simulink model "ME416_Autonomy_Model_Rollback2"  (R2025b)
settings: Solver=FixedStepAuto  StartTime=0.0  StopTime=240  RelTol=1e-3  EnableMultiTasking=on
PreLoadFcn:
  | driveparam
values from neighbouring files (symbols this model uses):
  alpha_w = 0.7    [driveparam.m]
  beta = Ts / (Ts + tau)    (= 0.166666666667)    [driveparam.m]
  enable_cmd = 1    [driveparam.m]
  estop_cmd = 0    [driveparam.m]
  K_lqr_w = dlqr(Ad_w, Bd_w, Qw, Rw)    [driveparam.m]
  L = 0.15    [driveparam.m]
  N = 4400    [driveparam.m]
  Nbar_lqr_w = (1 - Ad_w)/Bd_w + K_lqr_w    [driveparam.m]
  r = 0.03    [driveparam.m]
  Ts = 0.01    [driveparam.m]
  v_ref_cmd = 0    [driveparam.m]
  w_ref_cmd = 0.1    [driveparam.m]
undefined symbols (not defined in the file or in its folder): DiscIntNeverNeededParam, dspblkCoreblockFVToolHelper, gcbh
libraries: raspberrypiBasiclib x22, simulink x21, raspberrypiCommlib x19, slpidlib x2
(part 2 of 3)

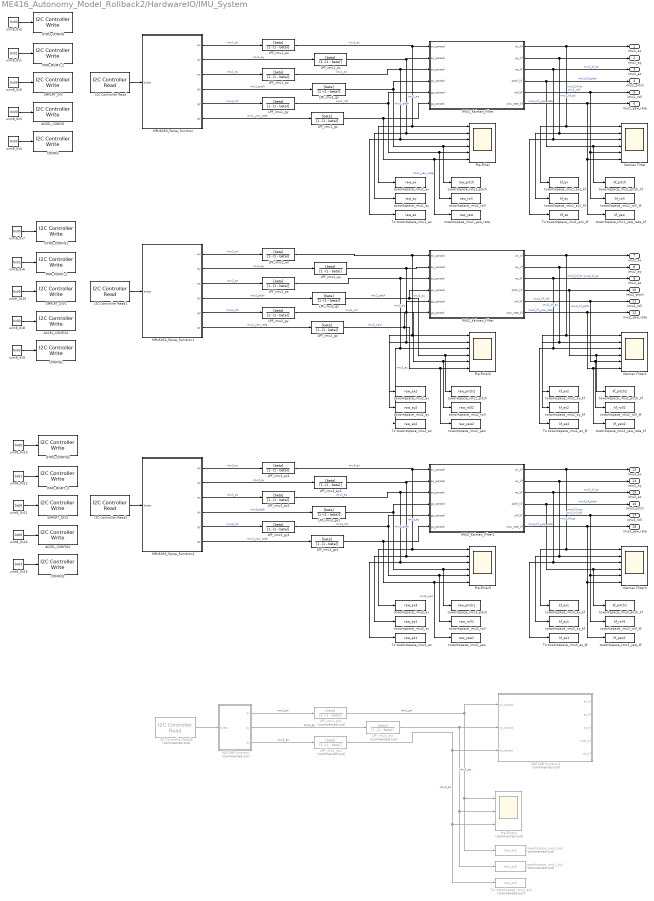
== system ME416_Autonomy_Model_Rollback2/HardwareIO/IMU_System ==
  ACCEL_CONFIG : raspberrypiCommlib/I2C Controller Write  BoardProperty=Pi 4 Model B  I2CModule=1  Mode=Master  SlaveAddress=0x68  SlaveByteOrder=BigEndian  Direction=Transmitter  RegisterAddressMode=on  RegisterAddress=0x1C  SlaveDataType=uint8  DataLength=1  NoAck=off  RepeatedStart=off  OutputStatus=off
  ACCEL_CONFIG1 : raspberrypiCommlib/I2C Controller Write  BoardProperty=Pi 4 Model B  I2CModule=0  Mode=Master  SlaveAddress=0x68  SlaveByteOrder=BigEndian  Direction=Transmitter  RegisterAddressMode=on  RegisterAddress=0x1C  SlaveDataType=uint8  DataLength=1  NoAck=off  RepeatedStart=off  OutputStatus=off
  ACCEL_CONFIG2 : raspberrypiCommlib/I2C Controller Write  BoardProperty=Pi 4 Model B  I2CModule=0  Mode=Master  SlaveAddress=0x69  SlaveByteOrder=BigEndian  Direction=Transmitter  RegisterAddressMode=on  RegisterAddress=0x1C  SlaveDataType=uint8  DataLength=1  NoAck=off  RepeatedStart=off  OutputStatus=off
  CONFIG : raspberrypiCommlib/I2C Controller Write  BoardProperty=Pi 4 Model B  I2CModule=1  Mode=Master  SlaveAddress=0x68  SlaveByteOrder=BigEndian  Direction=Transmitter  RegisterAddressMode=on  RegisterAddress=0x1A  SlaveDataType=uint8  DataLength=1  NoAck=off  RepeatedStart=off  OutputStatus=off
  CONFIG1 : raspberrypiCommlib/I2C Controller Write  BoardProperty=Pi 4 Model B  I2CModule=0  Mode=Master  SlaveAddress=0x68  SlaveByteOrder=BigEndian  Direction=Transmitter  RegisterAddressMode=on  RegisterAddress=0x1A  SlaveDataType=uint8  DataLength=1  NoAck=off  RepeatedStart=off  OutputStatus=off
  CONFIG2 : raspberrypiCommlib/I2C Controller Write  BoardProperty=Pi 4 Model B  I2CModule=0  Mode=Master  SlaveAddress=0x69  SlaveByteOrder=BigEndian  Direction=Transmitter  RegisterAddressMode=on  RegisterAddress=0x1A  SlaveDataType=uint8  DataLength=1  NoAck=off  RepeatedStart=off  OutputStatus=off
  GYRO_CONFIG : raspberrypiCommlib/I2C Controller Write  BoardProperty=Pi 4 Model B  I2CModule=1  Mode=Master  SlaveAddress=0x68  SlaveByteOrder=BigEndian  Direction=Transmitter  RegisterAddressMode=on  RegisterAddress=0x1B  SlaveDataType=uint8  DataLength=1  NoAck=off  RepeatedStart=off  OutputStatus=off
  GYRO_CONFIG1 : raspberrypiCommlib/I2C Controller Write  BoardProperty=Pi 4 Model B  I2CModule=0  Mode=Master  SlaveAddress=0x68  SlaveByteOrder=BigEndian  Direction=Transmitter  RegisterAddressMode=on  RegisterAddress=0x1B  SlaveDataType=uint8  DataLength=1  NoAck=off  RepeatedStart=off  OutputStatus=off
  GYRO_CONFIG2 : raspberrypiCommlib/I2C Controller Write  BoardProperty=Pi 4 Model B  I2CModule=0  Mode=Master  SlaveAddress=0x69  SlaveByteOrder=BigEndian  Direction=Transmitter  RegisterAddressMode=on  RegisterAddress=0x1B  SlaveDataType=uint8  DataLength=1  NoAck=off  RepeatedStart=off  OutputStatus=off
  I2C Controller Read : raspberrypiCommlib/I2C Controller Read  BoardProperty=Pi 4 Model B  I2CModule=1  Mode=Master  SlaveAddress=0x68  SlaveByteOrder=BigEndian  Direction=Receiver  RegisterAddressMode=on  RegisterAddress=0x3B  SlaveDataType=uint8  DataLength=14  NoAck=off  RepeatedStart=off  OutputStatus=off  SampleTime=0.01
  I2C Controller Read1 : raspberrypiCommlib/I2C Controller Read  BoardProperty=Pi 4 Model B  I2CModule=0  Mode=Master  SlaveAddress=0x68  SlaveByteOrder=BigEndian  Direction=Receiver  RegisterAddressMode=on  RegisterAddress=0x3B  SlaveDataType=uint8  DataLength=14  NoAck=off  RepeatedStart=off  OutputStatus=off  SampleTime=0.01
  I2C Controller Read2 : raspberrypiCommlib/I2C Controller Read  BoardProperty=Pi 4 Model B  I2CModule=0  Mode=Master  SlaveAddress=0x69  SlaveByteOrder=BigEndian  Direction=Receiver  RegisterAddressMode=on  RegisterAddress=0x3B  SlaveDataType=uint8  DataLength=14  NoAck=off  RepeatedStart=off  OutputStatus=off  SampleTime=0.01
  I2C Controller Read3 : raspberrypiCommlib/I2C Controller Read  Commented=on  BoardProperty=Pi 4 Model B  I2CModule=1  Mode=Master  SlaveAddress=0x1C  SlaveByteOrder=BigEndian  Direction=Receiver  RegisterAddressMode=on  RegisterAddress=0x01  SlaveDataType=uint8  DataLength=6  NoAck=off  RepeatedStart=off  OutputStatus=off  SampleTime=0.01
  IMU1_Kalman_Filter : MATLAB Function  TreatAsAtomicUnit=on
  IMU2_Kalman_Filter : MATLAB Function  TreatAsAtomicUnit=on
  IMU2_Kalman_Filter1 : MATLAB Function  TreatAsAtomicUnit=on
  Kalman Filter : Scope  NumInputPorts=6
      settings: ActiveDisplayYMinimum=-0.15082916961218429  ActiveDisplayYMaximum=0.016758796623576027
  Kalman Filter2 : Scope  NumInputPorts=6
      settings: ActiveDisplayYMinimum=-0.15082916961218429  ActiveDisplayYMaximum=0.016758796623576027  DataLoggingVariableName=ScopeData6
  Kalman Filter3 : Scope  NumInputPorts=6
      settings: ActiveDisplayYMinimum=-0.15082916961218429  ActiveDisplayYMaximum=0.016758796623576027  DataLoggingVariableName=ScopeData11
  LPF_imu1_ax : DiscreteTransferFcn  LoadFcn=dspblkCoreblockFVToolHelper(gcbh,'load');  Numerator=[beta]  Denominator=[1 -(1 - beta)]  SampleTime=Ts
      settings: CopyFcn=dspblkCoreblockFVToolHelper(gcbh,'copy');  DeleteFcn=dspblkCoreblockFVToolHelper(gcbh,'close');  ModelCloseFcn=dspblkCoreblockFVToolHelper(gcbh,'close');  PreSaveFcn=dspblkCoreblockFVToolHelper(gcbh,'presave');  PostSaveFcn=dspblkCoreblockFVToolHelper(gcbh,'postsave');  CloseFcn=dspblkCoreblockFVToolHelper(gcbh,'close');
  LPF_imu1_ax1 : DiscreteTransferFcn  Commented=on  LoadFcn=dspblkCoreblockFVToolHelper(gcbh,'load');  Numerator=[beta]  Denominator=[1 -(1 - beta)]  SampleTime=Ts
      settings: CopyFcn=dspblkCoreblockFVToolHelper(gcbh,'copy');  DeleteFcn=dspblkCoreblockFVToolHelper(gcbh,'close');  ModelCloseFcn=dspblkCoreblockFVToolHelper(gcbh,'close');  PreSaveFcn=dspblkCoreblockFVToolHelper(gcbh,'presave');  PostSaveFcn=dspblkCoreblockFVToolHelper(gcbh,'postsave');  CloseFcn=dspblkCoreblockFVToolHelper(gcbh,'close');
  LPF_imu1_ay : DiscreteTransferFcn  LoadFcn=dspblkCoreblockFVToolHelper(gcbh,'load');  Numerator=[beta]  Denominator=[1 -(1 - beta)]  SampleTime=Ts
      settings: CopyFcn=dspblkCoreblockFVToolHelper(gcbh,'copy');  DeleteFcn=dspblkCoreblockFVToolHelper(gcbh,'close');  ModelCloseFcn=dspblkCoreblockFVToolHelper(gcbh,'close');  PreSaveFcn=dspblkCoreblockFVToolHelper(gcbh,'presave');  PostSaveFcn=dspblkCoreblockFVToolHelper(gcbh,'postsave');  CloseFcn=dspblkCoreblockFVToolHelper(gcbh,'close');
  LPF_imu1_ay1 : DiscreteTransferFcn  Commented=on  LoadFcn=dspblkCoreblockFVToolHelper(gcbh,'load');  Numerator=[beta]  Denominator=[1 -(1 - beta)]  SampleTime=Ts
      settings: CopyFcn=dspblkCoreblockFVToolHelper(gcbh,'copy');  DeleteFcn=dspblkCoreblockFVToolHelper(gcbh,'close');  ModelCloseFcn=dspblkCoreblockFVToolHelper(gcbh,'close');  PreSaveFcn=dspblkCoreblockFVToolHelper(gcbh,'presave');  PostSaveFcn=dspblkCoreblockFVToolHelper(gcbh,'postsave');  CloseFcn=dspblkCoreblockFVToolHelper(gcbh,'close');
  LPF_imu1_az : DiscreteTransferFcn  LoadFcn=dspblkCoreblockFVToolHelper(gcbh,'load');  Numerator=[beta]  Denominator=[1 -(1 - beta)]  SampleTime=Ts
      settings: CopyFcn=dspblkCoreblockFVToolHelper(gcbh,'copy');  DeleteFcn=dspblkCoreblockFVToolHelper(gcbh,'close');  ModelCloseFcn=dspblkCoreblockFVToolHelper(gcbh,'close');  PreSaveFcn=dspblkCoreblockFVToolHelper(gcbh,'presave');  PostSaveFcn=dspblkCoreblockFVToolHelper(gcbh,'postsave');  CloseFcn=dspblkCoreblockFVToolHelper(gcbh,'close');
  LPF_imu1_az1 : DiscreteTransferFcn  Commented=on  LoadFcn=dspblkCoreblockFVToolHelper(gcbh,'load');  Numerator=[beta]  Denominator=[1 -(1 - beta)]  SampleTime=Ts
      settings: CopyFcn=dspblkCoreblockFVToolHelper(gcbh,'copy');  DeleteFcn=dspblkCoreblockFVToolHelper(gcbh,'close');  ModelCloseFcn=dspblkCoreblockFVToolHelper(gcbh,'close');  PreSaveFcn=dspblkCoreblockFVToolHelper(gcbh,'presave');  PostSaveFcn=dspblkCoreblockFVToolHelper(gcbh,'postsave');  CloseFcn=dspblkCoreblockFVToolHelper(gcbh,'close');
  LPF_imu1_gx : DiscreteTransferFcn  LoadFcn=dspblkCoreblockFVToolHelper(gcbh,'load');  Numerator=[beta]  Denominator=[1 -(1 - beta)]  SampleTime=Ts
      settings: CopyFcn=dspblkCoreblockFVToolHelper(gcbh,'copy');  DeleteFcn=dspblkCoreblockFVToolHelper(gcbh,'close');  ModelCloseFcn=dspblkCoreblockFVToolHelper(gcbh,'close');  PreSaveFcn=dspblkCoreblockFVToolHelper(gcbh,'presave');  PostSaveFcn=dspblkCoreblockFVToolHelper(gcbh,'postsave');  CloseFcn=dspblkCoreblockFVToolHelper(gcbh,'close');
  LPF_imu1_gy : DiscreteTransferFcn  LoadFcn=dspblkCoreblockFVToolHelper(gcbh,'load');  Numerator=[beta]  Denominator=[1 -(1 - beta)]  SampleTime=Ts
      settings: CopyFcn=dspblkCoreblockFVToolHelper(gcbh,'copy');  DeleteFcn=dspblkCoreblockFVToolHelper(gcbh,'close');  ModelCloseFcn=dspblkCoreblockFVToolHelper(gcbh,'close');  PreSaveFcn=dspblkCoreblockFVToolHelper(gcbh,'presave');  PostSaveFcn=dspblkCoreblockFVToolHelper(gcbh,'postsave');  CloseFcn=dspblkCoreblockFVToolHelper(gcbh,'close');
  LPF_imu1_gz : DiscreteTransferFcn  LoadFcn=dspblkCoreblockFVToolHelper(gcbh,'load');  Numerator=[beta]  Denominator=[1 -(1 - beta)]  SampleTime=Ts
      settings: CopyFcn=dspblkCoreblockFVToolHelper(gcbh,'copy');  DeleteFcn=dspblkCoreblockFVToolHelper(gcbh,'close');  ModelCloseFcn=dspblkCoreblockFVToolHelper(gcbh,'close');  PreSaveFcn=dspblkCoreblockFVToolHelper(gcbh,'presave');  PostSaveFcn=dspblkCoreblockFVToolHelper(gcbh,'postsave');  CloseFcn=dspblkCoreblockFVToolHelper(gcbh,'close');
  LPF_imu2_ax : DiscreteTransferFcn  LoadFcn=dspblkCoreblockFVToolHelper(gcbh,'load');  Numerator=[beta]  Denominator=[1 -(1 - beta)]  SampleTime=Ts
      settings: CopyFcn=dspblkCoreblockFVToolHelper(gcbh,'copy');  DeleteFcn=dspblkCoreblockFVToolHelper(gcbh,'close');  ModelCloseFcn=dspblkCoreblockFVToolHelper(gcbh,'close');  PreSaveFcn=dspblkCoreblockFVToolHelper(gcbh,'presave');  PostSaveFcn=dspblkCoreblockFVToolHelper(gcbh,'postsave');  CloseFcn=dspblkCoreblockFVToolHelper(gcbh,'close');
  LPF_imu2_ay : DiscreteTransferFcn  LoadFcn=dspblkCoreblockFVToolHelper(gcbh,'load');  Numerator=[beta]  Denominator=[1 -(1 - beta)]  SampleTime=Ts
      settings: CopyFcn=dspblkCoreblockFVToolHelper(gcbh,'copy');  DeleteFcn=dspblkCoreblockFVToolHelper(gcbh,'close');  ModelCloseFcn=dspblkCoreblockFVToolHelper(gcbh,'close');  PreSaveFcn=dspblkCoreblockFVToolHelper(gcbh,'presave');  PostSaveFcn=dspblkCoreblockFVToolHelper(gcbh,'postsave');  CloseFcn=dspblkCoreblockFVToolHelper(gcbh,'close');
  LPF_imu2_az : DiscreteTransferFcn  LoadFcn=dspblkCoreblockFVToolHelper(gcbh,'load');  Numerator=[beta]  Denominator=[1 -(1 - beta)]  SampleTime=Ts
      settings: CopyFcn=dspblkCoreblockFVToolHelper(gcbh,'copy');  DeleteFcn=dspblkCoreblockFVToolHelper(gcbh,'close');  ModelCloseFcn=dspblkCoreblockFVToolHelper(gcbh,'close');  PreSaveFcn=dspblkCoreblockFVToolHelper(gcbh,'presave');  PostSaveFcn=dspblkCoreblockFVToolHelper(gcbh,'postsave');  CloseFcn=dspblkCoreblockFVToolHelper(gcbh,'close');
  LPF_imu2_gx : DiscreteTransferFcn  LoadFcn=dspblkCoreblockFVToolHelper(gcbh,'load');  Numerator=[beta]  Denominator=[1 -(1 - beta)]  SampleTime=Ts
      settings: CopyFcn=dspblkCoreblockFVToolHelper(gcbh,'copy');  DeleteFcn=dspblkCoreblockFVToolHelper(gcbh,'close');  ModelCloseFcn=dspblkCoreblockFVToolHelper(gcbh,'close');  PreSaveFcn=dspblkCoreblockFVToolHelper(gcbh,'presave');  PostSaveFcn=dspblkCoreblockFVToolHelper(gcbh,'postsave');  CloseFcn=dspblkCoreblockFVToolHelper(gcbh,'close');
  LPF_imu2_gy : DiscreteTransferFcn  LoadFcn=dspblkCoreblockFVToolHelper(gcbh,'load');  Numerator=[beta]  Denominator=[1 -(1 - beta)]  SampleTime=Ts
      settings: CopyFcn=dspblkCoreblockFVToolHelper(gcbh,'copy');  DeleteFcn=dspblkCoreblockFVToolHelper(gcbh,'close');  ModelCloseFcn=dspblkCoreblockFVToolHelper(gcbh,'close');  PreSaveFcn=dspblkCoreblockFVToolHelper(gcbh,'presave');  PostSaveFcn=dspblkCoreblockFVToolHelper(gcbh,'postsave');  CloseFcn=dspblkCoreblockFVToolHelper(gcbh,'close');
  LPF_imu2_gz : DiscreteTransferFcn  LoadFcn=dspblkCoreblockFVToolHelper(gcbh,'load');  Numerator=[beta]  Denominator=[1 -(1 - beta)]  SampleTime=Ts
      settings: CopyFcn=dspblkCoreblockFVToolHelper(gcbh,'copy');  DeleteFcn=dspblkCoreblockFVToolHelper(gcbh,'close');  ModelCloseFcn=dspblkCoreblockFVToolHelper(gcbh,'close');  PreSaveFcn=dspblkCoreblockFVToolHelper(gcbh,'presave');  PostSaveFcn=dspblkCoreblockFVToolHelper(gcbh,'postsave');  CloseFcn=dspblkCoreblockFVToolHelper(gcbh,'close');
  LPF_imu3_ax1 : DiscreteTransferFcn  LoadFcn=dspblkCoreblockFVToolHelper(gcbh,'load');  Numerator=[beta]  Denominator=[1 -(1 - beta)]  SampleTime=Ts
      settings: CopyFcn=dspblkCoreblockFVToolHelper(gcbh,'copy');  DeleteFcn=dspblkCoreblockFVToolHelper(gcbh,'close');  ModelCloseFcn=dspblkCoreblockFVToolHelper(gcbh,'close');  PreSaveFcn=dspblkCoreblockFVToolHelper(gcbh,'presave');  PostSaveFcn=dspblkCoreblockFVToolHelper(gcbh,'postsave');  CloseFcn=dspblkCoreblockFVToolHelper(gcbh,'close');
  LPF_imu3_ay1 : DiscreteTransferFcn  LoadFcn=dspblkCoreblockFVToolHelper(gcbh,'load');  Numerator=[beta]  Denominator=[1 -(1 - beta)]  SampleTime=Ts
      settings: CopyFcn=dspblkCoreblockFVToolHelper(gcbh,'copy');  DeleteFcn=dspblkCoreblockFVToolHelper(gcbh,'close');  ModelCloseFcn=dspblkCoreblockFVToolHelper(gcbh,'close');  PreSaveFcn=dspblkCoreblockFVToolHelper(gcbh,'presave');  PostSaveFcn=dspblkCoreblockFVToolHelper(gcbh,'postsave');  CloseFcn=dspblkCoreblockFVToolHelper(gcbh,'close');
  LPF_imu3_az1 : DiscreteTransferFcn  LoadFcn=dspblkCoreblockFVToolHelper(gcbh,'load');  Numerator=[beta]  Denominator=[1 -(1 - beta)]  SampleTime=Ts
      settings: CopyFcn=dspblkCoreblockFVToolHelper(gcbh,'copy');  DeleteFcn=dspblkCoreblockFVToolHelper(gcbh,'close');  ModelCloseFcn=dspblkCoreblockFVToolHelper(gcbh,'close');  PreSaveFcn=dspblkCoreblockFVToolHelper(gcbh,'presave');  PostSaveFcn=dspblkCoreblockFVToolHelper(gcbh,'postsave');  CloseFcn=dspblkCoreblockFVToolHelper(gcbh,'close');
  LPF_imu3_gx1 : DiscreteTransferFcn  LoadFcn=dspblkCoreblockFVToolHelper(gcbh,'load');  Numerator=[beta]  Denominator=[1 -(1 - beta)]  SampleTime=Ts
      settings: CopyFcn=dspblkCoreblockFVToolHelper(gcbh,'copy');  DeleteFcn=dspblkCoreblockFVToolHelper(gcbh,'close');  ModelCloseFcn=dspblkCoreblockFVToolHelper(gcbh,'close');  PreSaveFcn=dspblkCoreblockFVToolHelper(gcbh,'presave');  PostSaveFcn=dspblkCoreblockFVToolHelper(gcbh,'postsave');  CloseFcn=dspblkCoreblockFVToolHelper(gcbh,'close');
  LPF_imu3_gy1 : DiscreteTransferFcn  LoadFcn=dspblkCoreblockFVToolHelper(gcbh,'load');  Numerator=[beta]  Denominator=[1 -(1 - beta)]  SampleTime=Ts
      settings: CopyFcn=dspblkCoreblockFVToolHelper(gcbh,'copy');  DeleteFcn=dspblkCoreblockFVToolHelper(gcbh,'close');  ModelCloseFcn=dspblkCoreblockFVToolHelper(gcbh,'close');  PreSaveFcn=dspblkCoreblockFVToolHelper(gcbh,'presave');  PostSaveFcn=dspblkCoreblockFVToolHelper(gcbh,'postsave');  CloseFcn=dspblkCoreblockFVToolHelper(gcbh,'close');
  LPF_imu3_gz1 : DiscreteTransferFcn  LoadFcn=dspblkCoreblockFVToolHelper(gcbh,'load');  Numerator=[beta]  Denominator=[1 -(1 - beta)]  SampleTime=Ts
      settings: CopyFcn=dspblkCoreblockFVToolHelper(gcbh,'copy');  DeleteFcn=dspblkCoreblockFVToolHelper(gcbh,'close');  ModelCloseFcn=dspblkCoreblockFVToolHelper(gcbh,'close');  PreSaveFcn=dspblkCoreblockFVToolHelper(gcbh,'presave');  PostSaveFcn=dspblkCoreblockFVToolHelper(gcbh,'postsave');  CloseFcn=dspblkCoreblockFVToolHelper(gcbh,'close');
  MATLAB Function : MATLAB Function  Commented=on  TreatAsAtomicUnit=on
  MATLAB Function1 : MATLAB Function  Commented=on  TreatAsAtomicUnit=on
  MPU6050_Parse_Function : MATLAB Function  TreatAsAtomicUnit=on
  MPU6050_Parse_Function1 : MATLAB Function  TreatAsAtomicUnit=on
  MPU6050_Parse_Function2 : MATLAB Function  TreatAsAtomicUnit=on
  PWR_MGMT_1 : raspberrypiCommlib/I2C Controller Write  BoardProperty=Pi 4 Model B  I2CModule=1  Mode=Master  SlaveAddress=0x68  SlaveByteOrder=BigEndian  Direction=Transmitter  RegisterAddressMode=on  RegisterAddress=0x6B  SlaveDataType=uint8  DataLength=1  NoAck=off  RepeatedStart=off  OutputStatus=off
  PWR_MGMT_2 : raspberrypiCommlib/I2C Controller Write  BoardProperty=Pi 4 Model B  I2CModule=0  Mode=Master  SlaveAddress=0x68  SlaveByteOrder=BigEndian  Direction=Transmitter  RegisterAddressMode=on  RegisterAddress=0x6B  SlaveDataType=uint8  DataLength=1  NoAck=off  RepeatedStart=off  OutputStatus=off
  PWR_MGMT_3 : raspberrypiCommlib/I2C Controller Write  BoardProperty=Pi 4 Model B  I2CModule=0  Mode=Master  SlaveAddress=0x69  SlaveByteOrder=BigEndian  Direction=Transmitter  RegisterAddressMode=on  RegisterAddress=0x6B  SlaveDataType=uint8  DataLength=1  NoAck=off  RepeatedStart=off  OutputStatus=off
  Pre-Filter : Scope  NumInputPorts=6
      settings: ActiveDisplayYMinimum=-0.68608023128352935  ActiveDisplayYMaximum=0.076231136809281022  DataLoggingVariableName=ScopeData5
  Pre-Filter1 : Scope  Commented=on  NumInputPorts=3
      settings: ActiveDisplayYMinimum=-0.68608023128352935  ActiveDisplayYMaximum=0.076231136809281022  DataLoggingVariableName=ScopeData13
  Pre-Filter2 : Scope  NumInputPorts=6
      settings: ActiveDisplayYMinimum=-0.68608023128352935  ActiveDisplayYMaximum=0.076231136809281022  DataLoggingVariableName=ScopeData10
  Pre-Filter3 : Scope  NumInputPorts=6
      settings: ActiveDisplayYMinimum=-0.68608023128352935  ActiveDisplayYMaximum=0.076231136809281022  DataLoggingVariableName=ScopeData12
  SMPLRT_DIV : raspberrypiCommlib/I2C Controller Write  BoardProperty=Pi 4 Model B  I2CModule=1  Mode=Master  SlaveAddress=0x68  SlaveByteOrder=BigEndian  Direction=Transmitter  RegisterAddressMode=on  RegisterAddress=0x19  SlaveDataType=uint8  DataLength=1  NoAck=off  RepeatedStart=off  OutputStatus=off
  SMPLRT_DIV1 : raspberrypiCommlib/I2C Controller Write  BoardProperty=Pi 4 Model B  I2CModule=0  Mode=Master  SlaveAddress=0x68  SlaveByteOrder=BigEndian  Direction=Transmitter  RegisterAddressMode=on  RegisterAddress=0x19  SlaveDataType=uint8  DataLength=1  NoAck=off  RepeatedStart=off  OutputStatus=off
  SMPLRT_DIV2 : raspberrypiCommlib/I2C Controller Write  BoardProperty=Pi 4 Model B  I2CModule=0  Mode=Master  SlaveAddress=0x69  SlaveByteOrder=BigEndian  Direction=Transmitter  RegisterAddressMode=on  RegisterAddress=0x19  SlaveDataType=uint8  DataLength=1  NoAck=off  RepeatedStart=off  OutputStatus=off
  To toworkspace_imu1_az : ToWorkspace  VariableName=raw_az  SampleTime=-1
  To toworkspace_imu1_az1 : ToWorkspace  Commented=on  VariableName=raw_az3  SampleTime=-1
  To toworkspace_imu1_az1_kf : ToWorkspace  VariableName=kf_az  SampleTime=-1
  To toworkspace_imu2_az : ToWorkspace  VariableName=raw_az2  SampleTime=-1
  To toworkspace_imu2_az_kf : ToWorkspace  VariableName=kf_az2  SampleTime=-1
  To toworkspace_imu3_az : ToWorkspace  VariableName=raw_az1  SampleTime=-1
  To toworkspace_imu3_az_kf : ToWorkspace  VariableName=kf_az1  SampleTime=-1
  toworkspace_imu1_ax : ToWorkspace  VariableName=raw_ax  SampleTime=-1
  toworkspace_imu1_ax1 : ToWorkspace  Commented=on  VariableName=raw_ax1  SampleTime=-1
  toworkspace_imu1_ax1_kf : ToWorkspace  VariableName=kf_ax  SampleTime=-1
  toworkspace_imu1_ay : ToWorkspace  VariableName=raw_ay  SampleTime=-1
  toworkspace_imu1_ay1 : ToWorkspace  Commented=on  VariableName=raw_ay3  SampleTime=-1
  toworkspace_imu1_ay1_kf : ToWorkspace  VariableName=kf_ay  SampleTime=-1
  toworkspace_imu1_pitch : ToWorkspace  VariableName=raw_pitch  SampleTime=-1
  toworkspace_imu1_pitch_kf : ToWorkspace  VariableName=kf_pitch  SampleTime=-1
  toworkspace_imu1_roll : ToWorkspace  VariableName=raw_roll  SampleTime=-1
  toworkspace_imu1_roll_kf : ToWorkspace  VariableName=kf_roll  SampleTime=-1
  toworkspace_imu1_yaw_rate : ToWorkspace  VariableName=raw_yaw  SampleTime=-1
  toworkspace_imu1_yaw_rate_kf : ToWorkspace  VariableName=kf_yaw  SampleTime=-1
  toworkspace_imu2_ax : ToWorkspace  VariableName=raw_ax2  SampleTime=-1
  toworkspace_imu2_ax_kf : ToWorkspace  VariableName=kf_ax2  SampleTime=-1
  toworkspace_imu2_ay : ToWorkspace  VariableName=raw_ay2  SampleTime=-1
  toworkspace_imu2_ay_kf : ToWorkspace  VariableName=kf_ay2  SampleTime=-1
  toworkspace_imu2_pitch : ToWorkspace  VariableName=raw_pitch2  SampleTime=-1
  toworkspace_imu2_pitch_kf : ToWorkspace  VariableName=kf_pitch2  SampleTime=-1
  toworkspace_imu2_roll : ToWorkspace  VariableName=raw_roll2  SampleTime=-1
  toworkspace_imu2_roll_kf : ToWorkspace  VariableName=kf_roll2  SampleTime=-1
  toworkspace_imu2_yaw : ToWorkspace  VariableName=raw_yaw2  SampleTime=-1
  toworkspace_imu2_yaw_rate_kf : ToWorkspace  VariableName=kf_yaw2  SampleTime=-1
  toworkspace_imu3_ax : ToWorkspace  VariableName=raw_ax3  SampleTime=-1
  toworkspace_imu3_ax_kf : ToWorkspace  VariableName=kf_ax1  SampleTime=-1
  toworkspace_imu3_ay : ToWorkspace  VariableName=raw_ay1  SampleTime=-1
  toworkspace_imu3_ay_kf : ToWorkspace  VariableName=kf_ay1  SampleTime=-1
  toworkspace_imu3_pitch : ToWorkspace  VariableName=raw_pitch1  SampleTime=-1
  toworkspace_imu3_pitch_kf : ToWorkspace  VariableName=kf_pitch1  SampleTime=-1
  toworkspace_imu3_roll : ToWorkspace  VariableName=raw_roll1  SampleTime=-1
  toworkspace_imu3_roll_kf : ToWorkspace  VariableName=kf_roll1  SampleTime=-1
  toworkspace_imu3_yaw : ToWorkspace  VariableName=raw_yaw1  SampleTime=-1
  toworkspace_imu3_yaw_kf : ToWorkspace  VariableName=kf_yaw1  SampleTime=-1
  uint8_0x1 : Constant  Value=0x01  OutDataTypeStr=uint8
  uint8_0x10 : Constant  Value=0x09  OutDataTypeStr=uint8
  uint8_0x11 : Constant  Value=0x09  OutDataTypeStr=uint8
  uint8_0x12 : Constant  Value=0x01  OutDataTypeStr=uint8
  uint8_0x{2..3,7..8,13..14} (6 alike) : Constant  Value=0x00  OutDataTypeStr=uint8
  uint8_0x15 : Constant  Value=0x03  OutDataTypeStr=uint8
  uint8_0x4 : Constant  Value=0x03  OutDataTypeStr=uint8
  uint8_0x5 : Constant  Value=0x09  OutDataTypeStr=uint8
  uint8_0x6 : Constant  Value=0x01  OutDataTypeStr=uint8
  uint8_0x9 : Constant  Value=0x03  OutDataTypeStr=uint8
  imu1_ax : Outport
  imu1_ay : Outport  Port=2
  imu1_az : Outport  Port=3
  imu1_pitch : Outport  Port=4
  imu1_roll : Outport  Port=5
  imu1_yaw_rate : Outport  Port=6
  imu2_ax : Outport  Port=7
  imu2_ay : Outport  Port=8
  imu2_az : Outport  Port=9
  imu2_pitch : Outport  Port=10
  imu2_roll : Outport  Port=11
  imu2_yaw_rate : Outport  Port=12
  imu3_ax : Outport  Port=13
  imu3_ay : Outport  Port=14
  imu3_az : Outport  Port=15
  imu3_pitch : Outport  Port=16
  imu3_roll : Outport  Port=17
  imu3_yaw_rate : Outport  Port=18
  wires:
  LPF_imu1_gz/1 -> IMU1_Kalman_Filter/6(gz_parsed), Pre-Filter/6, toworkspace_imu1_yaw_rate/1  "imu1_yaw_rate"
  LPF_imu1_gy/1 -> IMU1_Kalman_Filter/5(gy_parsed), Pre-Filter/5, toworkspace_imu1_roll/1  "imu1_roll"
  IMU1_Kalman_Filter/4(pitch_kf) -> imu1_pitch/1, toworkspace_imu1_pitch_kf/1, Kalman Filter/4  "imu1_kf_pitch"
  LPF_imu1_gx/1 -> IMU1_Kalman_Filter/4(gx_parsed), toworkspace_imu1_pitch/1, Pre-Filter/4  "imu1_pitch"
  LPF_imu1_ax/1 -> IMU1_Kalman_Filter/1(ax_parsed), toworkspace_imu1_ax/1, Pre-Filter/1  "imu1_ax"
  IMU1_Kalman_Filter/3(az_kf) -> imu1_az/1, To toworkspace_imu1_az1_kf/1, Kalman Filter/3  "imu1_kf_az"
  LPF_imu1_az/1 -> IMU1_Kalman_Filter/3(az_parsed), To toworkspace_imu1_az/1, Pre-Filter/3  "imu1_az"
  IMU1_Kalman_Filter/1(ax_kf) -> imu1_ax/1, toworkspace_imu1_ax1_kf/1, Kalman Filter/1  "imu1_kf_ax"
  IMU1_Kalman_Filter/6(yaw_rate_kf) -> imu1_yaw_rate/1, toworkspace_imu1_yaw_rate_kf/1, Kalman Filter/6  "imu1_kf_yaw_rate"
  IMU1_Kalman_Filter/2(ay_kf) -> imu1_ay/1, toworkspace_imu1_ay1_kf/1, Kalman Filter/2  "imu1_kf_ay"
  MPU6050_Parse_Function/6(gz) -> LPF_imu1_gz/1  "imu1_yaw_rate"
  LPF_imu1_ay/1 -> IMU1_Kalman_Filter/2(ay_parsed), toworkspace_imu1_ay/1, Pre-Filter/2  "imu1_ay"
  MPU6050_Parse_Function/5(gy) -> LPF_imu1_gy/1  "imu1_roll"
  IMU1_Kalman_Filter/5(roll_kf) -> imu1_roll/1, Kalman Filter/5, toworkspace_imu1_roll_kf/1  "imu1_roll"
  MPU6050_Parse_Function/3(az) -> LPF_imu1_az/1  "imu1_az"
  I2C Controller Read/1 -> MPU6050_Parse_Function/1(bytes)
  MPU6050_Parse_Function/1(ax) -> LPF_imu1_ax/1  "imu1_ax"
  MPU6050_Parse_Function/2(ay) -> LPF_imu1_ay/1  "imu1_ay"
  MPU6050_Parse_Function/4(gx) -> LPF_imu1_gx/1  "imu1_pitch"
  LPF_imu2_gz/1 -> IMU2_Kalman_Filter/6(gz_parsed), Pre-Filter2/6, toworkspace_imu2_yaw/1  "imu2_yaw"
  LPF_imu2_gy/1 -> IMU2_Kalman_Filter/5(gy_parsed), Pre-Filter2/5, toworkspace_imu2_roll/1  "imu2_roll"
  MPU6050_Parse_Function1/4(gx) -> LPF_imu2_gx/1  "imu2_pitch"
  MPU6050_Parse_Function1/2(ay) -> LPF_imu2_ay/1  "imu2_ay"
  I2C Controller Read1/1 -> MPU6050_Parse_Function1/1(bytes)
  MPU6050_Parse_Function1/1(ax) -> LPF_imu2_ax/1  "imu2_ax"
  MPU6050_Parse_Function1/3(az) -> LPF_imu2_az/1  "imu2_az"
  MPU6050_Parse_Function1/5(gy) -> LPF_imu2_gy/1  "imu2_roll"
  LPF_imu2_ay/1 -> IMU2_Kalman_Filter/2(ay_parsed), toworkspace_imu2_ay/1, Pre-Filter2/2  "imu2_ay"
  IMU2_Kalman_Filter/5(roll_kf) -> imu2_roll/1, Kalman Filter2/5, toworkspace_imu2_roll_kf/1  "imu2_kf_roll"
  IMU2_Kalman_Filter/2(ay_kf) -> imu2_ay/1, toworkspace_imu2_ay_kf/1, Kalman Filter2/2  "imu2_kf_ay"
  MPU6050_Parse_Function1/6(gz) -> LPF_imu2_gz/1  "imu2_yaw_rate"
  IMU2_Kalman_Filter/3(az_kf) -> imu2_az/1, To toworkspace_imu2_az_kf/1, Kalman Filter2/3  "imu2_kf_az"
  IMU2_Kalman_Filter/6(yaw_rate_kf) -> imu2_yaw_rate/1, toworkspace_imu2_yaw_rate_kf/1, Kalman Filter2/6  "imu2_kf_yaw_rate"
  IMU2_Kalman_Filter/1(ax_kf) -> imu2_ax/1, toworkspace_imu2_ax_kf/1, Kalman Filter2/1  "imu2_kf_ax"
  LPF_imu2_gx/1 -> IMU2_Kalman_Filter/4(gx_parsed), toworkspace_imu2_pitch/1, Pre-Filter2/4  "imu2_pitch"
  LPF_imu2_ax/1 -> IMU2_Kalman_Filter/1(ax_parsed), toworkspace_imu2_ax/1, Pre-Filter2/1  "imu2_ax"
  LPF_imu2_az/1 -> IMU2_Kalman_Filter/3(az_parsed), To toworkspace_imu2_az/1, Pre-Filter2/3  "imu2_az"
  IMU2_Kalman_Filter/4(pitch_kf) -> imu2_pitch/1, toworkspace_imu2_pitch_kf/1, Kalman Filter2/4  "imu2_kf_pitch"
  MPU6050_Parse_Function2/4(gx) -> LPF_imu3_gx1/1  "imu3_pitch"
  MPU6050_Parse_Function2/1(ax) -> LPF_imu3_ax1/1  "imu3_ax"
  IMU2_Kalman_Filter1/1(ax_kf) -> imu3_ax/1, toworkspace_imu3_ax_kf/1, Kalman Filter3/1  "imu3_kf_ax"
  MPU6050_Parse_Function2/2(ay) -> LPF_imu3_ay1/1  "imu3_ay"
  IMU2_Kalman_Filter1/3(az_kf) -> imu3_az/1, To toworkspace_imu3_az_kf/1, Kalman Filter3/3  "imu3_kf_az"
  LPF_imu3_gx1/1 -> IMU2_Kalman_Filter1/4(gx_parsed), toworkspace_imu3_pitch/1, Pre-Filter3/4  "imu3_pitch"
  IMU2_Kalman_Filter1/2(ay_kf) -> imu3_ay/1, toworkspace_imu3_ay_kf/1, Kalman Filter3/2  "imu3_kf_ay"
  I2C Controller Read2/1 -> MPU6050_Parse_Function2/1(bytes)
  LPF_imu3_ay1/1 -> IMU2_Kalman_Filter1/2(ay_parsed), toworkspace_imu3_ay/1, Pre-Filter3/2  "imu3_ay"
  LPF_imu3_az1/1 -> IMU2_Kalman_Filter1/3(az_parsed), To toworkspace_imu3_az/1, Pre-Filter3/3  "imu3_az"
  LPF_imu3_gy1/1 -> IMU2_Kalman_Filter1/5(gy_parsed), Pre-Filter3/5, toworkspace_imu3_roll/1  "imu3_roll"
  IMU2_Kalman_Filter1/5(roll_kf) -> imu3_roll/1, Kalman Filter3/5, toworkspace_imu3_roll_kf/1  "imu3_kf_roll"
  MPU6050_Parse_Function2/6(gz) -> LPF_imu3_gz1/1  "imu3_yaw_rate"
  LPF_imu3_ax1/1 -> IMU2_Kalman_Filter1/1(ax_parsed), toworkspace_imu3_ax/1, Pre-Filter3/1  "imu3_ax"
  IMU2_Kalman_Filter1/6(yaw_rate_kf) -> imu3_yaw_rate/1, toworkspace_imu3_yaw_kf/1, Kalman Filter3/6  "imu3_kf_yaw_rate"
  MPU6050_Parse_Function2/3(az) -> LPF_imu3_az1/1  "imu3_az"
  IMU2_Kalman_Filter1/4(pitch_kf) -> imu3_pitch/1, toworkspace_imu3_pitch_kf/1, Kalman Filter3/4  "imu3_kf_pitch"
  LPF_imu3_gz1/1 -> IMU2_Kalman_Filter1/6(gz_parsed), Pre-Filter3/6, toworkspace_imu3_yaw/1  "imu3_yaw"
  MPU6050_Parse_Function2/5(gy) -> LPF_imu3_gy1/1  "imu3_roll"
  LPF_imu1_az1/1 -> MATLAB Function1/3(az_parsed), To toworkspace_imu1_az1/1, Pre-Filter1/3  "imu1_az"
  MATLAB Function/3(az) -> LPF_imu1_az1/1  "imu1_az"
  MATLAB Function/2(ay) -> LPF_imu1_ay1/1  "imu1_ay"
  MATLAB Function/1(ax) -> LPF_imu1_ax1/1  "imu1_ax"
  I2C Controller Read3/1 -> MATLAB Function/1(bytes)
  LPF_imu1_ax1/1 -> toworkspace_imu1_ax1/1, Pre-Filter1/1, MATLAB Function1/1(ax_parsed)  "imu1_ax"
  LPF_imu1_ay1/1 -> MATLAB Function1/2(ay_parsed), toworkspace_imu1_ay1/1, Pre-Filter1/2  "imu1_ay"
  uint8_0x5/1 -> SMPLRT_DIV/1
  uint8_0x3/1 -> ACCEL_CONFIG/1
  uint8_0x4/1 -> CONFIG/1
  uint8_0x2/1 -> GYRO_CONFIG/1
  uint8_0x1/1 -> PWR_MGMT_1/1
  uint8_0x6/1 -> PWR_MGMT_2/1
  uint8_0x8/1 -> ACCEL_CONFIG1/1
  uint8_0x10/1 -> SMPLRT_DIV1/1
  uint8_0x7/1 -> GYRO_CONFIG1/1
  uint8_0x9/1 -> CONFIG1/1
  uint8_0x15/1 -> CONFIG2/1
  uint8_0x11/1 -> SMPLRT_DIV2/1
  uint8_0x13/1 -> GYRO_CONFIG2/1
  uint8_0x14/1 -> ACCEL_CONFIG2/1
  uint8_0x12/1 -> PWR_MGMT_3/1

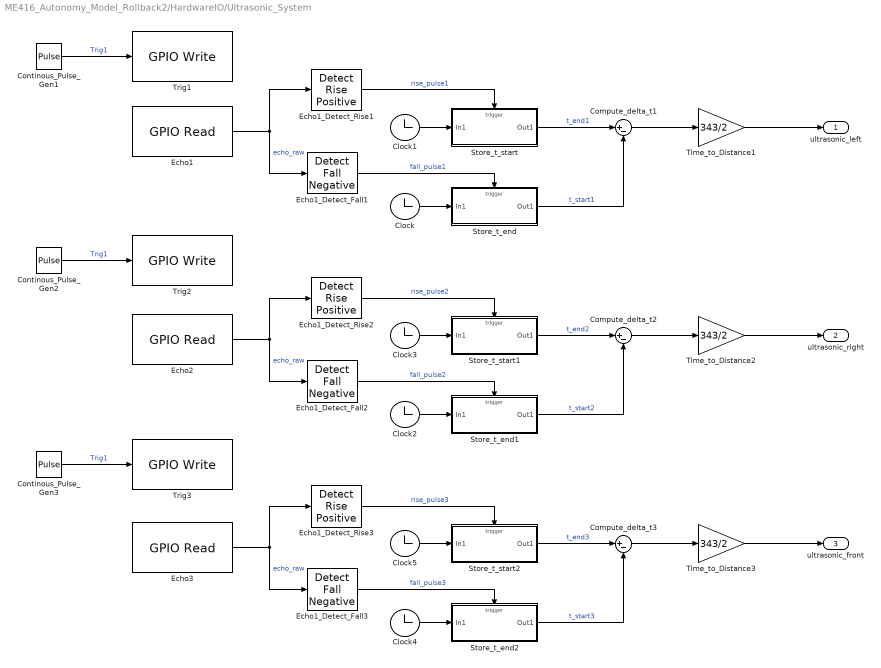
== system ME416_Autonomy_Model_Rollback2/HardwareIO/Ultrasonic_System ==
  Clock{,1..5} (6 alike) : Clock
  Compute_delta_t1 : Sum  Inputs=|+-
  Compute_delta_t2 : Sum  Inputs=|+-
  Compute_delta_t3 : Sum  Inputs=|+-
  Continous_Pulse_Gen1 : DiscretePulseGenerator  PulseType=Time based  Period=0.06  PulseWidth=0.00001
  Continous_Pulse_Gen2 : DiscretePulseGenerator  PulseType=Time based  Period=0.06  PulseWidth=0.00001
  Continous_Pulse_Gen3 : DiscretePulseGenerator  PulseType=Time based  Period=0.06  PulseWidth=0.00001
  Echo1 : raspberrypiBasiclib/GPIO Read  BoardProperty=Pi 4 Model B  gpio=9  SampleTime=-1  blockPlatform=Raspberry Pi  PinNumber=4  board=[]  direction=[]  internalResistor=[]
  Echo1_Detect_Fall1 : simulink/Logic and Bit Operations/Detect Fall Negative  vinit=0  OutDataTypeStr=boolean
  Echo1_Detect_Fall2 : simulink/Logic and Bit Operations/Detect Fall Negative  vinit=0  OutDataTypeStr=boolean
  Echo1_Detect_Fall3 : simulink/Logic and Bit Operations/Detect Fall Negative  vinit=0  OutDataTypeStr=boolean
  Echo1_Detect_Rise1 : simulink/Logic and Bit Operations/Detect Rise Positive  vinit=0  OutDataTypeStr=boolean
  Echo1_Detect_Rise2 : simulink/Logic and Bit Operations/Detect Rise Positive  vinit=0  OutDataTypeStr=boolean
  Echo1_Detect_Rise3 : simulink/Logic and Bit Operations/Detect Rise Positive  vinit=0  OutDataTypeStr=boolean
  Echo2 : raspberrypiBasiclib/GPIO Read  BoardProperty=Pi 4 Model B  gpio=26  SampleTime=-1  blockPlatform=Raspberry Pi  PinNumber=4  board=[]  direction=[]  internalResistor=[]
  Echo3 : raspberrypiBasiclib/GPIO Read  BoardProperty=Pi 4 Model B  gpio=6  SampleTime=-1  blockPlatform=Raspberry Pi  PinNumber=4  board=[]  direction=[]  internalResistor=[]
  Store_t_end : Subsystem  TreatAsAtomicUnit=on
  Store_t_end1 : Subsystem  TreatAsAtomicUnit=on
  Store_t_end2 : Subsystem  TreatAsAtomicUnit=on
  Store_t_start : Subsystem  TreatAsAtomicUnit=on
  Store_t_start1 : Subsystem  TreatAsAtomicUnit=on
  Store_t_start2 : Subsystem  TreatAsAtomicUnit=on
  Time_to_Distance1 : Gain  Gain=343/2
  Time_to_Distance2 : Gain  Gain=343/2
  Time_to_Distance3 : Gain  Gain=343/2
  Trig1 : raspberrypiBasiclib/GPIO Write  BoardProperty=Pi 4 Model B  gpio=10  blockPlatform=Raspberry Pi  PinNumber=17  board=[]  direction=[]
  Trig2 : raspberrypiBasiclib/GPIO Write  BoardProperty=Pi 4 Model B  gpio=11  blockPlatform=Raspberry Pi  PinNumber=17  board=[]  direction=[]
  Trig3 : raspberrypiBasiclib/GPIO Write  BoardProperty=Pi 4 Model B  gpio=5  blockPlatform=Raspberry Pi  PinNumber=17  board=[]  direction=[]
  ultrasonic_left : Outport
  ultrasonic_right : Outport  Port=2
  ultrasonic_front : Outport  Port=3
  wires:
  Compute_delta_t1/1 -> Time_to_Distance1/1
  Echo1_Detect_Rise3/1 -> Store_t_start2/Trigger  "rise_pulse3"
  Echo1_Detect_Fall1/1 -> Store_t_end/Trigger  "fall_pulse1"
  Time_to_Distance3/1 -> ultrasonic_front/1
  Store_t_end1/1(Out1) -> Compute_delta_t2/2  "t_start2"
  Compute_delta_t3/1 -> Time_to_Distance3/1
  Clock2/1 -> Store_t_end1/1(In1)
  Clock4/1 -> Store_t_end2/1(In1)
  Time_to_Distance2/1 -> ultrasonic_right/1
  Store_t_end2/1(Out1) -> Compute_delta_t3/2  "t_start3"
  Store_t_start/1(Out1) -> Compute_delta_t1/1  "t_end1"
  Compute_delta_t2/1 -> Time_to_Distance2/1
  Echo3/1 -> Echo1_Detect_Fall3/1, Echo1_Detect_Rise3/1  "echo_raw"
  Echo1_Detect_Fall2/1 -> Store_t_end1/Trigger  "fall_pulse2"
  Continous_Pulse_Gen3/1 -> Trig3/1  "Trig1"
  Clock5/1 -> Store_t_start2/1(In1)
  Store_t_start1/1(Out1) -> Compute_delta_t2/1  "t_end2"
  Store_t_start2/1(Out1) -> Compute_delta_t3/1  "t_end3"
  Continous_Pulse_Gen2/1 -> Trig2/1  "Trig1"
  Echo1_Detect_Fall3/1 -> Store_t_end2/Trigger  "fall_pulse3"
  Echo1_Detect_Rise1/1 -> Store_t_start/Trigger  "rise_pulse1"
  Echo1/1 -> Echo1_Detect_Fall1/1, Echo1_Detect_Rise1/1  "echo_raw"
  Time_to_Distance1/1 -> ultrasonic_left/1
  Continous_Pulse_Gen1/1 -> Trig1/1  "Trig1"
  Echo1_Detect_Rise2/1 -> Store_t_start1/Trigger  "rise_pulse2"
  Echo2/1 -> Echo1_Detect_Fall2/1, Echo1_Detect_Rise2/1  "echo_raw"
  Clock3/1 -> Store_t_start1/1(In1)
  Clock1/1 -> Store_t_start/1(In1)
  Store_t_end/1(Out1) -> Compute_delta_t1/2  "t_start1"
  Clock/1 -> Store_t_end/1(In1)

== system ME416_Autonomy_Model_Rollback2/ArmControl (Jacobian + PID Joints)/HoldAndStabilize/latch_pitch_ref ==
  imu3_pitch : Inport
  Trigger : TriggerPort  VariantControl=(inherit)
  pitch_ref : Outport
  wires:
  imu3_pitch/1 -> pitch_ref/1

== system ME416_Autonomy_Model_Rollback2/ArmControl (Jacobian + PID Joints)/JointController/Latch_Actuate_Start_Time ==
  In1 : Inport
  Trigger : TriggerPort  VariantControl=(inherit)
  Out1 : Outport
  wires:
  In1/1 -> Out1/1

== system ME416_Autonomy_Model_Rollback2/ArmControl (Jacobian + PID Joints)/JointController/Latch_Post_Start_Time ==
  In1 : Inport
  Trigger : TriggerPort  VariantControl=(inherit)
  Out1 : Outport
  wires:
  In1/1 -> Out1/1

== system ME416_Autonomy_Model_Rollback2/DriveControl (PID, LQR, IMU, Encoder, DC Motors)/StateEstimate/PoseEstimator ==
  v_meas : Inport
  w_meas : Inport  Port=2
  Product : Product
  Product1 : Product
  Trigonometric Function : Trigonometry
  Trigonometric Function1 : Trigonometry  Operator=cos
  theta_integrator : DiscreteIntegrator  SampleTime=Ts  ICPrevOutput=DiscIntNeverNeededParam  ICPrevScaledInput=DiscIntNeverNeededParam
  x_integrator : DiscreteIntegrator  SampleTime=Ts  ICPrevOutput=DiscIntNeverNeededParam  ICPrevScaledInput=DiscIntNeverNeededParam
  y_integrator : DiscreteIntegrator  SampleTime=Ts  ICPrevOutput=DiscIntNeverNeededParam  ICPrevScaledInput=DiscIntNeverNeededParam
  theta_hat : Outport
  x_hat : Outport  Port=2
  x_dot : Outport  Port=3
  y_hat : Outport  Port=4
  y_dot : Outport  Port=5
  wires:
  Trigonometric Function/1 -> Product/1  "sin_theta_hat"
  theta_integrator/1 -> Trigonometric Function/1, theta_hat/1, Trigonometric Function1/1
  Trigonometric Function1/1 -> Product1/1  "cos_theta_hat"
  v_meas/1 -> Product/2, Product1/2
  Product/1 -> y_dot/1, y_integrator/1
  Product1/1 -> x_dot/1, x_integrator/1
  y_integrator/1 -> y_hat/1
  x_integrator/1 -> x_hat/1
  w_meas/1 -> theta_integrator/1

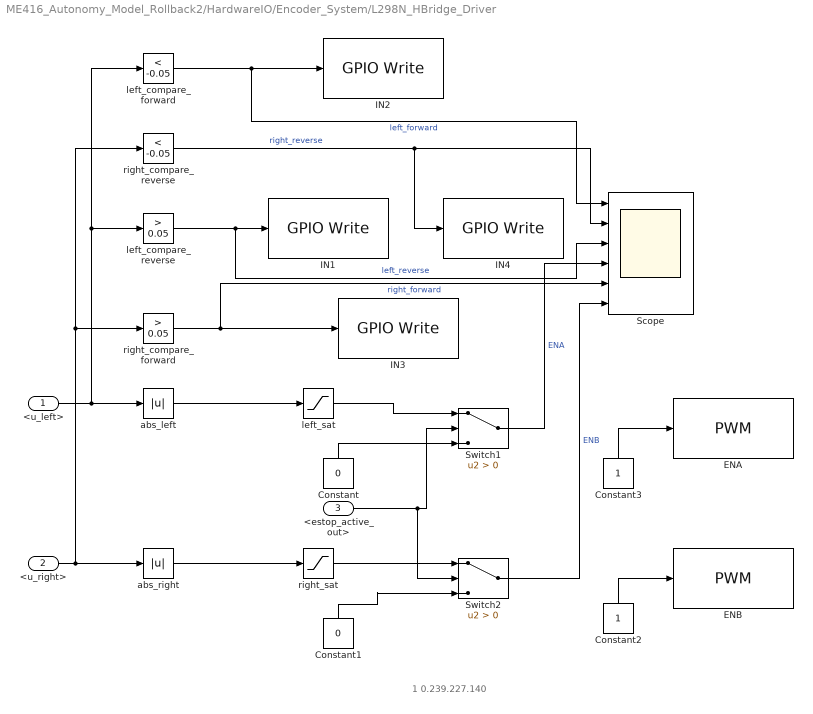
== system ME416_Autonomy_Model_Rollback2/HardwareIO/Encoder_System/L298N_HBridge_Driver ==
  note: 1 0.239.227.140
  <u_left> : Inport
  <u_right> : Inport  Port=2
  <estop_active_out> : Inport  Port=3
  Constant : Constant  Value=0
  Constant1 : Constant  Value=0
  Constant2 : Constant
  Constant3 : Constant
  ENA : raspberrypiBasiclib/PWM  board=Pi 4 Model B  Pin_=14  Frequency=500  blockPlatform=Raspberry Pi
  ENB : raspberrypiBasiclib/PWM  board=Pi 4 Model B  Pin_=15  Frequency=500  blockPlatform=Raspberry Pi
  IN1 : raspberrypiBasiclib/GPIO Write  BoardProperty=Pi 4 Model B  gpio=24  blockPlatform=Raspberry Pi  PinNumber=17  board=Pi 4 Model B  direction=Output
  IN2 : raspberrypiBasiclib/GPIO Write  BoardProperty=Pi 4 Model B  gpio=23  blockPlatform=Raspberry Pi  PinNumber=17  board=Pi 4 Model B  direction=Output
  IN3 : raspberrypiBasiclib/GPIO Write  BoardProperty=Pi 4 Model B  gpio=25  blockPlatform=Raspberry Pi  PinNumber=17  board=Pi 4 Model B  direction=Output
  IN4 : raspberrypiBasiclib/GPIO Write  BoardProperty=Pi 4 Model B  gpio=8  blockPlatform=Raspberry Pi  PinNumber=17  board=Pi 4 Model B  direction=Output
  Scope : Scope  NumInputPorts=6
      settings: ActiveDisplayYMinimum=-1  ActiveDisplayYMaximum=1  DataLoggingVariableName=ScopeData9
  Switch1 : Switch  Criteria=u2 > Threshold  SaturateOnIntegerOverflow=off  InputSameDT=off
  Switch2 : Switch  Criteria=u2 > Threshold  SaturateOnIntegerOverflow=off  InputSameDT=off
  abs_left : Abs  SaturateOnIntegerOverflow=off
  abs_right : Abs  SaturateOnIntegerOverflow=off
  left_compare_forward : simulink/Logic and Bit Operations/Compare To Constant  relop=<  const=-0.05  OutDataTypeStr=boolean
  left_compare_reverse : simulink/Logic and Bit Operations/Compare To Constant  relop=>  const=0.05  OutDataTypeStr=boolean
  left_sat : Saturate  UpperLimit=1  LowerLimit=0
  right_compare_forward : simulink/Logic and Bit Operations/Compare To Constant  relop=>  const=0.05  OutDataTypeStr=boolean
  right_compare_reverse : simulink/Logic and Bit Operations/Compare To Constant  relop=<  const=-0.05  OutDataTypeStr=boolean
  right_sat : Saturate  UpperLimit=1  LowerLimit=0
  wires:
  <u_right>/1 -> right_compare_forward/1, right_compare_reverse/1, abs_right/1
  Constant1/1 -> Switch2/3
  <u_left>/1 -> left_compare_reverse/1, left_compare_forward/1, abs_left/1
  right_compare_forward/1 -> Scope/5, IN3/1  "right_forward"
  left_compare_forward/1 -> Scope/1, IN2/1  "left_forward"
  Switch1/1 -> Scope/4  "ENA"
  left_compare_reverse/1 -> Scope/3, IN1/1  "left_reverse"
  abs_left/1 -> left_sat/1
  abs_right/1 -> right_sat/1
  right_compare_reverse/1 -> Scope/2, IN4/1  "right_reverse"
  left_sat/1 -> Switch1/1
  Constant/1 -> Switch1/3
  <estop_active_out>/1 -> Switch2/2, Switch1/2
  right_sat/1 -> Switch2/1
  Switch2/1 -> Scope/6  "ENB"
  Constant2/1 -> ENB/1
  Constant3/1 -> ENA/1

== system ME416_Autonomy_Model_Rollback2/HardwareIO/Encoder_System/LeftEncoderQuadrature ==
  Constant : Constant
  Constant1 : Constant  Value=-1
  Logical Operator : Logic  AllPortsSameDT=off  OutDataTypeStr=boolean
  Logical Operator1 : Logic  Operator=NOT  AllPortsSameDT=off  OutDataTypeStr=boolean
  Product : Product
  Scope : Scope  NumInputPorts=2
      settings: DataLoggingVariableName=ScopeData7
  Sum : Sum  Inputs=|++
  Switch : Switch  Criteria=u2 > Threshold  SaturateOnIntegerOverflow=off  InputSameDT=off
  count_delay : UnitDelay  SampleTime=0.001  HasFrameUpgradeWarning=on
  enc_left_phaseA : raspberrypiBasiclib/GPIO Read  BoardProperty=Pi 4 Model B  gpio=12  SampleTime=0.001  blockPlatform=Raspberry Pi  PinNumber=4  board=Pi 4 Model B  direction=Input  internalResistor=Off
  enc_left_phaseB : raspberrypiBasiclib/GPIO Read  BoardProperty=Pi 4 Model B  gpio=16  SampleTime=0.001  blockPlatform=Raspberry Pi  PinNumber=4  board=Pi 4 Model B  direction=Input  internalResistor=Off
  phaseA_delay : UnitDelay  SampleTime=0.001  HasFrameUpgradeWarning=on
  enc_left_ticks : Outport
  wires:
  enc_left_phaseB/1 -> Switch/2, Scope/2
  Constant/1 -> Switch/1
  Logical Operator1/1 -> Logical Operator/2
  Constant1/1 -> Switch/3
  enc_left_phaseA/1 -> phaseA_delay/1, Logical Operator/1, Scope/1
  Logical Operator/1 -> Product/1  "A_rise"
  Switch/1 -> Product/2  "dir_step"
  Sum/1 -> count_delay/1, enc_left_ticks/1
  count_delay/1 -> Sum/2
  Product/1 -> Sum/1  "delta_count"
  phaseA_delay/1 -> Logical Operator1/1

== system ME416_Autonomy_Model_Rollback2/HardwareIO/Encoder_System/RightEncoderQuadrature ==
  Constant : Constant
  Constant1 : Constant  Value=-1
  Logical Operator : Logic  AllPortsSameDT=off  OutDataTypeStr=boolean
  Logical Operator1 : Logic  Operator=NOT  AllPortsSameDT=off  OutDataTypeStr=boolean
  Product : Product
  Scope : Scope  NumInputPorts=2
      settings: ActiveDisplayYMinimum=-0.12499999999999997  ActiveDisplayYMaximum=1.125  DataLoggingVariableName=ScopeData8
  Sum : Sum  Inputs=|++
  Switch : Switch  Threshold=0.5  SaturateOnIntegerOverflow=off  InputSameDT=off
  count_delay : UnitDelay  SampleTime=0.001  HasFrameUpgradeWarning=on
  enc_right_phaseA : raspberrypiBasiclib/GPIO Read  BoardProperty=Pi 4 Model B  gpio=20  SampleTime=0.001  blockPlatform=Raspberry Pi  PinNumber=4  board=Model B+  direction=Input  internalResistor=Off
  enc_right_phaseB : raspberrypiBasiclib/GPIO Read  BoardProperty=Pi 4 Model B  gpio=21  SampleTime=0.001  blockPlatform=Raspberry Pi  PinNumber=4  board=Model B+  direction=Input  internalResistor=Off
  phaseA_delay : UnitDelay  SampleTime=0.001  HasFrameUpgradeWarning=on
  enc_right_ticks : Outport
  wires:
  Switch/1 -> Product/2  "dir_step"
  Constant1/1 -> Switch/3
  Constant/1 -> Switch/1
  Sum/1 -> count_delay/1, enc_right_ticks/1
  Logical Operator1/1 -> Logical Operator/2
  Logical Operator/1 -> Product/1  "A_rise"
  enc_right_phaseB/1 -> Scope/2, Switch/2
  enc_right_phaseA/1 -> phaseA_delay/1, Logical Operator/1, Scope/1
  count_delay/1 -> Sum/2
  Product/1 -> Sum/1  "delta_count"
  phaseA_delay/1 -> Logical Operator1/1

== system ME416_Autonomy_Model_Rollback2/HardwareIO/Ultrasonic_System/Store_t_end ==
  In1 : Inport
  Trigger : TriggerPort  VariantControl=(inherit)
  Out1 : Outport
  wires:
  In1/1 -> Out1/1

== system ME416_Autonomy_Model_Rollback2/HardwareIO/Ultrasonic_System/Store_t_end1 ==
  In1 : Inport
  Trigger : TriggerPort  VariantControl=(inherit)
  Out1 : Outport
  wires:
  In1/1 -> Out1/1

== system ME416_Autonomy_Model_Rollback2/HardwareIO/Ultrasonic_System/Store_t_end2 ==
  In1 : Inport
  Trigger : TriggerPort  VariantControl=(inherit)
  Out1 : Outport
  wires:
  In1/1 -> Out1/1

== system ME416_Autonomy_Model_Rollback2/HardwareIO/Ultrasonic_System/Store_t_start ==
  In1 : Inport
  Trigger : TriggerPort  VariantControl=(inherit)
  Out1 : Outport
  wires:
  In1/1 -> Out1/1

== system ME416_Autonomy_Model_Rollback2/HardwareIO/Ultrasonic_System/Store_t_start1 ==
  In1 : Inport
  Trigger : TriggerPort  VariantControl=(inherit)
  Out1 : Outport
  wires:
  In1/1 -> Out1/1

== system ME416_Autonomy_Model_Rollback2/HardwareIO/Ultrasonic_System/Store_t_start2 ==
  In1 : Inport
  Trigger : TriggerPort  VariantControl=(inherit)
  Out1 : Outport
  wires:
  In1/1 -> Out1/1

== stateflow chart ME416_Autonomy_Model_Rollback2/Supervisor (FSM)1/FSM ==
  state OFF
    during:
    is_poweron = false;
    is_post = false;
    is_search = false;
    is_chase = false;
    is_compute = false;
    is_actuate = false;
    drive_stop_cmd = true;
  state DONE
    during:
    is_poweron = true;
    is_post = false;
    is_search = false;
    is_chase = false;
    is_compute = false;
    is_actuate = false;
    drive_stop_cmd = true;
  state POST
    during:
    is_poweron = true;
    is_post = true;
    is_search = false;
    is_chase = false;
    is_compute = false;
    is_actuate = false;
    drive_stop_cmd = true;
  state ESTOP
    during:
    is_poweron = false;
    is_post = false;
    is_search = false;
    is_chase = false;
    is_compute = false;
    is_actuate = false;
    drive_stop_cmd = true;
  state ACTUATE
    during:
    is_poweron = true;
    is_post = false;
    is_search = false;
    is_chase = false;
    is_compute = false;
    is_actuate = true;
    drive_stop_cmd = true;
  state SEARCH
    during:
    is_poweron = true;
    is_post = false;
    is_search = true;
    is_chase = false;
    is_compute = false;
    is_actuate = false;
    drive_stop_cmd = false;
  state CHASE
    during:
    is_poweron = true;
    is_post = false;
    is_search = false;
    is_chase = true;
    is_compute = false;
    is_actuate = false;
    drive_stop_cmd = false;
  state COMPUTE_IK
    during:
    is_poweron = true;
    is_post = false;
    is_search = false;
    is_chase = false;
    is_compute = true;
    is_actuate = false;
    drive_stop_cmd = true;
  (default) -> OFF
  OFF -> POST [order 1] : [power_on && ~estop]
  OFF -> ESTOP [order 2] : [estop]
  DONE -> ESTOP : [estop]
  POST -> ESTOP [order 2] : [estop]
  POST -> SEARCH [order 1] : [post_done]
  ACTUATE -> DONE [order 1] : [actuation_done]
  SEARCH -> ESTOP [order 2] : [estop]
  ACTUATE -> ESTOP [order 2] : [estop]
  CHASE -> ESTOP [order 2] : [estop]
  COMPUTE_IK -> ESTOP [order 2] : [estop]
  SEARCH -> CHASE [order 1] : [tag_found]
  COMPUTE_IK -> ACTUATE [order 1] : [ik_done && ik_valid]
  CHASE -> COMPUTE_IK [order 1] : [target_reached]
  data: power_on input; post_done input; tag_found input; target_reached input; ik_done input; ik_valid input; actuation_done input; estop input; is_poweron output boolean; is_post output boolean; is_search output boolean; is_chase output boolean; is_compute output boolean; is_actuate output boolean; drive_stop_cmd output boolean

== matlab function ME416_Autonomy_Model_Rollback2/HardwareIO/IMU_System/IMU2_Kalman_Filter1 ==
  data: ax_parsed input; ax_kf output; ay_parsed input; az_parsed input; gx_parsed input; ay_kf output; az_kf output; pitch_kf output; roll_kf output; yaw_rate_kf output; gy_parsed input; gz_parsed input
function [ax_kf, ay_kf, az_kf, pitch_kf, roll_kf, yaw_rate_kf] = imu_kalman_filter(ax_parsed, ay_parsed, az_parsed, gx_parsed, gy_parsed, gz_parsed)
%#codegen
% Simple 1D Kalman smoothing filter for IMU signals
%
% Inputs:
%   ax, ay, az   -> accelerometer in g
%   gx, gy, gz   -> gyro in rad/sa
%
% Outputs:
%   ax_f, ay_f, az_f     -> filtered accel
%   pitch_f, roll_f      -> filtered angles from accel
%   yaw_rate_f           -> filtered yaw rate from gyro z

% Persistent states for each filtered signal
persistent x_ax_parsed p_ax_parsed
persistent x_ay_parsed p_ay_parsed
persistent x_az_parsed p_az_parsed
persistent x_pitch p_pitch
persistent x_roll p_roll
persistent x_yaw p_yaw

% Tunable Kalman parameters
% Lower q = smoother/slower
% Lower r = trusts measurement more
q_acc = 0.001; r_acc = 0.2;
q_ang = 0.001; r_ang = 0.2;
q_yaw = 0.001; r_yaw = 0.3;

% Compute raw roll/pitch from accelerometer
roll_meas  = atan2(ay_parsed, az_parsed);
pitch_meas = atan2(-ax_parsed, sqrt(ay_parsed^2 + az_parsed^2));

% Initialize on first run
if isempty(x_ax_parsed)
    x_ax_parsed = ax_parsed;      p_ax_parsed = 1.0;
    x_ay_parsed = ay_parsed;      p_ay_parsed = 1.0;
    x_az_parsed = az_parsed;      p_az_parsed = 1.0;

    x_roll  = roll_meas;    p_roll  = 1.0;
    x_pitch = pitch_meas;   p_pitch = 1.0;

    x_yaw = gz_parsed;      p_yaw = 1.0;
end

% Filter accel channels
[x_ax_parsed, p_ax_parsed] = kalman_update(x_ax_parsed, p_ax_parsed, ax_parsed, q_acc, r_acc);
[x_ay_parsed, p_ay_parsed] = kalman_update(x_ay_parsed, p_ay_parsed, ay_parsed, q_acc, r_acc);
[x_az_parsed, p_az_parsed] = kalman_update(x_az_parsed, p_az_parsed, az_parsed, q_acc, r_acc);

% Filter roll/pitch angles
[x_roll, p_roll]   = kalman_update(x_roll, p_roll, roll_meas, q_ang, r_ang);
[x_pitch, p_pitch] = kalman_update(x_pitch, p_pitch, pitch_meas, q_ang, r_ang);

% Filter yaw rate (gyro z)
[x_yaw, p_yaw] = kalman_update(x_yaw, p_yaw, gz_parsed, q_yaw, r_yaw);

% Outputs
ax_kf = x_ax_parsed;
ay_kf = x_ay_parsed;
az_kf = x_az_parsed;

roll_kf     = x_roll;
pitch_kf    = x_pitch;
yaw_rate_kf = x_yaw;

end

function [x, p] = kalman_update(x, p, z, q, r)
% 1D Kalman filter update

% Prediction
p = p + q;

% Correction
k = p / (p + r);
x = x + k * (z - x);
p = (1 - k) * p;

end

== matlab function ME416_Autonomy_Model_Rollback2/HardwareIO/IMU_System/MPU6050_Parse_Function2 ==
  data: bytes input; ax output; ay output; az output; gx output; gy output; gz output
function [ax, ay, az, gx, gy, gz] = parse_mpu6050(bytes)
%#codegen
% bytes: 14x1 uint8 from MPU6050 starting at 0x3B

ax_raw = combineSigned(bytes(1),  bytes(2));
ay_raw = combineSigned(bytes(3),  bytes(4));
az_raw = combineSigned(bytes(5),  bytes(6));

gx_raw = combineSigned(bytes(9),  bytes(10));
gy_raw = combineSigned(bytes(11), bytes(12));
gz_raw = combineSigned(bytes(13), bytes(14));

% Scale assuming accel +/-2g, gyro +/-250 deg/s
ax = double(ax_raw) / 16384.0;
ay = double(ay_raw) / 16384.0;
az = double(az_raw) / 16384.0;

gx = double(gx_raw) / 131.0 * (pi / 180.0);
gy = double(gy_raw) / 131.0 * (pi / 180.0);
gz = double(gz_raw) / 131.0 * (pi / 180.0);

end

function x = combineSigned(hi, lo)
% hi, lo are uint8
u = bitor(bitshift(uint16(hi), 8), uint16(lo));

if u >= 32768
    x = int16(int32(u) - 65536);
else
    x = int16(u);
end
end

== matlab function ME416_Autonomy_Model_Rollback2/HardwareIO/IMU_System/MATLAB Function ==
  data: bytes input; ax output; ay output; az output
function [ax, ay, az] = parse_mma8451(bytes)
%#codegen
% bytes: 6x1 uint8 from MMA8451 starting at 0x01

ax_raw = combine14BitSigned(bytes(1), bytes(2));
ay_raw = combine14BitSigned(bytes(3), bytes(4));
az_raw = combine14BitSigned(bytes(5), bytes(6));

% Scale assuming accel +/-2g range (4096 counts/g)
ax = double(ax_raw) / 4096.0;
ay = double(ay_raw) / 4096.0;
az = double(az_raw) / 4096.0;
end

function x = combine14BitSigned(hi, lo)
% hi, lo are uint8
u = bitor(bitshift(uint16(hi), 8), uint16(lo));

% Handle two's complement for the 16-bit combined value
if u >= 32768
    signed_16 = int16(int32(u) - 65536);
else
    signed_16 = int16(u);
end

% Shift right by 2 to extract the left-justified 14-bit value
x = bitshift(signed_16, -2);
end
